simulink model "SF051A_SnsrOffsLrng"  (R2013b)
settings: Solver=FixedStepDiscrete  SolverMode=SingleTasking  StartTime=0.0  StopTime=1  FixedStep=0.002  RelTol=1e-3
undefined symbols (not defined in the file): ARCHGLBPRM_10MILLISEC_SEC_F32, ARCHGLBPRM_2MILLISEC_SEC_F32, ARCHGLBPRM_2PI_ULS_F32, ARCHGLBPRM_FLOATZEROTHD_ULS_F32, ARCHGLBPRM_PIOVER180_ULS_F32, CNV100MICROSECTOMILLISEC_MILLISECPERCNT_F32, CNV100MICROSECTOSEC_SECPERCNT_F32, COVRAMTRXNIT_ULS_F32, HWAUTHYTHD_ULS_F32, HWTQLRNGSTSLRND_CNT_U08, HWTQLRNGSTSNEGOFFS_CNT_U08, HWTQLRNGSTSNOTLRND_CNT_U08, HWTQLRNGSTSPOSOFFS_CNT_U08, HWTQLRNGSTSZEROOFFS_CNT_U08, HWTQLRNGTMRHILIM_SEC_F32, IDYMTRX_ULS_F32, IVS10MS_ULSPERSEC_F32, LRNGFILTICON_ULS_F32, NvmGetErrSts1, ONE_ULS_F32, SnsrOffsLrnd, SnsrOffsLrngFctEna, SnsrOffsLrngHwAgLrngDrvgDstThd, SnsrOffsLrngHwAgLrngEna, SnsrOffsLrngHwAgLrngHwVelThd, SnsrOffsLrngHwAgLrngSysTqThd, SnsrOffsLrngHwAgLrngSysTqThdMed, SnsrOffsLrngHwAgLrngSysTqThdTrustd, SnsrOffsLrngHwAgLrngSysTqThdWide, SnsrOffsLrngHwAgLrngTi, SnsrOffsLrngHwAgLrngVehSpdThd, SnsrOffsLrngHwAgLrngYawOffsDbnd, SnsrOffsLrngHwAgLrngYawRateThd, SnsrOffsLrngHwAgOffsLim, SnsrOffsLrngHwTqLrngEna, SnsrOffsLrngHwTqLrngEnaTiThd, SnsrOffsLrngHwTqLrngHwAgDbnd, SnsrOffsLrngHwTqLrngHwAgThd, SnsrOffsLrngHwTqLrngHwTqThd, SnsrOffsLrngHwTqLrngHwTqZeroOffsThd, SnsrOffsLrngHwTqLrngHwVelThd, SnsrOffsLrngHwTqLrngMeasTi, SnsrOffsLrngHwTqLrngMeasTiScar, SnsrOffsLrngHwTqLrngSampleImbThd1, SnsrOffsLrngHwTqLrngSampleImbThd2, SnsrOffsLrngHwTqLrngSampleThd1, SnsrOffsLrngHwTqLrngSampleThd2, SnsrOffsLrngHwTqLrngTiWghtCoeff, SnsrOffsLrngHwTqLrngVehSpdThd, SnsrOffsLrngHwTqOffsLim, SnsrOffsLrngSampleCntForHwTqLrngRst, SnsrOffsLrngTqInpDetnPwrEstimnThd, SnsrOffsLrngTqInpDetnSinGenrAmp, SnsrOffsLrngTqInpDetnSinGenrFrq, SnsrOffsLrngTqInpDetnStg1FilGain, SnsrOffsLrngTqInpDetnStg1WinSize, SnsrOffsLrngTqInpDetnStg2FilGainCen, SnsrOffsLrngTqInpDetnStg2FilGainDwn, SnsrOffsLrngTqInpDetnStg2FilGainUp, SnsrOffsLrngTqInpDetnStg2WinSize ... (+15)
libraries: Fil x34, FixdToFloat x17, FloatToFixd x16, NxtrLim x15, simulink x12, NxtrAbslt x12, NxtrNvM x8, NxtrMin x5, NxtrMath x3
(part 9 of 11)

== system SF051A_SnsrOffsLrng/SnsrOffsLrng/SnsrOffsLrngPer1/Learning/ForgettingFactor/ResetHwTqLrng/GetRefTmr100MicroSec32bit ==
  note: 1 count = 100 uSec
  note: seconds
  note: microseconds
  note: counts
  note: Wrap-to-zero
  note: GetRefTmr100MicroSec32bit
  note: Created Aug 18, 2015
      | Modified Oct 21, 2015
      | Modified Oct 30, 2015
      | Kevin Derry
  CopyRight2 : Subsystem  Description=|  mask(Copyright Information){none=on}
      | Copyright info block.                                               
      |                                                                     
      | Place copyright information at the top of every subsystem in design.
      mask prompts: none "No parameters"
      mask help: Place copyright information at the top of every subsystem in design.
      mask Display:
      | NxtrConf = 'Nexteer Confidential';
      | 
      | sys = bdroot; %handle for the current model ("system")
      | first = get_param(sys,'Created');
      | if(isempty(first))
      |     first = datestr(now,'yyyy');
      | else
      |     first = first(end-3:end);  %year is last four digits
      | end
      | 
      | last = get_param(sys,'LastModifiedDate');
      | if isempty(last)
      |     last = datestr(now,'yyyy');
      | else
      |     last = last(end-3:end);
      | end
      | 
      | if strcmp(first,last)
      |     fprintf('%s -- Copyright %s Nexteer',NxtrConf,first)
      | else
      |     fprintf('%s -- %s%s- %s Nexteer',NxtrConf,char(169),first,last)
      | end
  Count per uSec : Constant  Value=0.01
  Data Store Read1 : DataStoreRead  DataStoreName=SimnTi
  Data Type Conversion1 : DataTypeConversion  OutDataTypeStr=uint32
  Divide1 : Product  Inputs=**
  Divide2 : Product  Inputs=*/
  Max Counts : Constant  Value=2^32-1
  Product1 : Product
  Product2 : Product
  Rounding : Rounding
  Subtract1 : Sum  Inputs=+-
  uSec per Sec : Constant  Value=1000000
  RefTmr : Outport
  wires:
  Product2/1 -> Subtract1/2
  Subtract1/1 -> Data Type Conversion1/1
  Rounding/1 -> Product2/1
  Divide2/1 -> Rounding/1
  Max Counts/1 -> Divide2/2, Product2/2
  Divide1/1 -> Divide2/1, Subtract1/1
  Product1/1 -> Divide1/1
  Count per uSec/1 -> Divide1/2
  uSec per Sec/1 -> Product1/2
  Data Type Conversion1/1 -> RefTmr/1
  Data Store Read1/1 -> Product1/1

== system SF051A_SnsrOffsLrng/SnsrOffsLrng/SnsrOffsLrngPer1/Learning/ForgettingFactor/ResetHwTqLrng/Subsystem5 ==

== system SF051A_SnsrOffsLrng/SnsrOffsLrng/SnsrOffsLrngPer1/Learning/Recursive Least Square Regression/Calculate Covariance Matrix/Subsystem5 ==

== system SF051A_SnsrOffsLrng/SnsrOffsLrng/SnsrOffsLrngPer1/Learning/Recursive Least Square Regression/Calculate K Vector/Subsystem5 ==

== system SF051A_SnsrOffsLrng/SnsrOffsLrng/SnsrOffsLrngPer1/Learning/Recursive Least Square Regression/Update beta_k/Subsystem5 ==

== system SF051A_SnsrOffsLrng/SnsrOffsLrng/SnsrOffsLrngPer1/Learning/ValidityCheck/DecideOutputs/HwTrqNotLearnt ==
  Action Port : ActionPort  ActionType=else
  Constant1 : Constant  Value=false  OutDataTypeStr=boolean
      settings: AttributesFormatString=%<OutDataTypeStr>
  Constant3 : Constant  Value=HWTQLRNGSTSNOTLRND_CNT_U08  OutDataTypeStr=uint8
  Subsystem5 : Subsystem  Description=|  mask(Copyright Information){none=on}
      | Copyright info block.                                               
      |                                                                     
      | Place copyright information at the top of every subsystem in design.
      mask prompts: none "No parameters"
      mask help: Place copyright information at the top of every subsystem in design.
      mask Display:
      | NxtrConf = 'Nexteer Confidential';
      | 
      | sys = bdroot; %handle for the current model ("system")
      | first = get_param(sys,'Created');
      | first = first(end-3:end);  %year is last four digits
      | 
      | last = get_param(sys,'LastModifiedDate');
      | if isempty(last)
      |     last = datestr(now,'yyyy');
      | else
      |     last = last(end-3:end);
      | end
      | 
      | if strcmp(first,last)
      |     fprintf('%s -- Copyright %s Nexteer',NxtrConf,first)
      | else
      |     fprintf('%s -- %s%s- %s Nexteer',NxtrConf,char(169),first,last)
      | end
  LrngSts : Outport
  EstimnVld : Outport  Port=2
  wires:
  Constant3/1 -> LrngSts/1
  Constant1/1 -> EstimnVld/1

== system SF051A_SnsrOffsLrng/SnsrOffsLrng/SnsrOffsLrngPer1/Learning/ValidityCheck/DecideOutputs/HwTrqOffsetLearnt ==
  Action Port : ActionPort  ActionType=then
  Constant1 : Constant  Value=true  OutDataTypeStr=boolean
      settings: AttributesFormatString=%<OutDataTypeStr>
  Constant3 : Constant  Value=HWTQLRNGSTSLRND_CNT_U08  OutDataTypeStr=uint8
  Subsystem5 : Subsystem  Description=|  mask(Copyright Information){none=on}
      | Copyright info block.                                               
      |                                                                     
      | Place copyright information at the top of every subsystem in design.
      mask prompts: none "No parameters"
      mask help: Place copyright information at the top of every subsystem in design.
      mask Display:
      | NxtrConf = 'Nexteer Confidential';
      | 
      | sys = bdroot; %handle for the current model ("system")
      | first = get_param(sys,'Created');
      | first = first(end-3:end);  %year is last four digits
      | 
      | last = get_param(sys,'LastModifiedDate');
      | if isempty(last)
      |     last = datestr(now,'yyyy');
      | else
      |     last = last(end-3:end);
      | end
      | 
      | if strcmp(first,last)
      |     fprintf('%s -- Copyright %s Nexteer',NxtrConf,first)
      | else
      |     fprintf('%s -- %s%s- %s Nexteer',NxtrConf,char(169),first,last)
      | end
  LrngSts : Outport
  EstimnVld : Outport  Port=2
  wires:
  Constant1/1 -> EstimnVld/1
  Constant3/1 -> LrngSts/1

== system SF051A_SnsrOffsLrng/SnsrOffsLrng/SnsrOffsLrngPer1/Learning/ValidityCheck/DecideOutputs/Pos//Neg//Zero Offset Status Selector ==
  note: It selects the TOCStatus based on the value of the
      | estimated HwTrq Offset.
  note: TOCStatus
      | 0 = HwTrq NotLearned
      | 1 = Positive HwTrq Offset
      | 2 = Negative HwTrqOffset
      | 3 = Zero HwTrq Offset
      | 4 = HwTrq Offset Learned
  DriftEstimnOnCentr : Inport  RequirementInfo={'linktype_rmi_doors' '0000babd (/E-STEER Core/SubSystem Specifications/Application Functions/SF051A Sensor Offset Learning)' '#SF051A_186' 'true' 'REQ:SF051A_186' '' ; 'linktype_rmi_doors' '0000babd (/E-STEER Core/SubSystem Specifications/Application Functions/SF051A Sensor Offset Learning)' '#SF051A_195' 'true' 'REQ:SF051A_195' '' ; 'linktype_rmi_doors' '0000babd (/E-STEER Core/SubSystem Specifications/Application Functions/SF051A Sensor Offset Learning)' '#SF051A_194' 'true' 'REQ:SF051A_194' '' } %GIDa_29c46742_0190_4134_8ec7_44363e312a28
  Action Port : ActionPort  ActionType=elseif
  1_Positive HwTrq Offset : Subsystem  RequirementInfo={'linktype_rmi_doors' '0000babd (/E-STEER Core/SubSystem Specifications/Application Functions/SF051A Sensor Offset Learning)' '#SF051A_186' 'true' 'REQ:SF051A_186' '' } %GIDa_941a9e58_f1f3_40f2_8b3e_1b09aead3b41  TreatAsAtomicUnit=on
  2_Negative HwTrq Offset : Subsystem  RequirementInfo={'linktype_rmi_doors' '0000babd (/E-STEER Core/SubSystem Specifications/Application Functions/SF051A Sensor Offset Learning)' '#SF051A_195' 'true' 'REQ:SF051A_195' '' } %GIDa_c6d6cb28_240d_4435_ac45_3133f97fc59c  TreatAsAtomicUnit=on
  3_Zero HwTrq Offset : Subsystem  RequirementInfo={'linktype_rmi_doors' '0000babd (/E-STEER Core/SubSystem Specifications/Application Functions/SF051A Sensor Offset Learning)' '#SF051A_194' 'true' 'REQ:SF051A_194' '' } %GIDa_2db23fb9_9ed6_47ae_a299_df8f3702bd6f  TreatAsAtomicUnit=on
  Constant3 : Constant  Value=false  OutDataTypeStr=boolean
      settings: AttributesFormatString=%<OutDataTypeStr>
  Constant4 : Constant  RequirementInfo={'linktype_rmi_doors' '0000babd (/E-STEER Core/SubSystem Specifications/Application Functions/SF051A Sensor Offset Learning)' '#SF051A_186' 'true' 'REQ:SF051A_186' '' ; 'linktype_rmi_doors' '0000babd (/E-STEER Core/SubSystem Specifications/Application Functions/SF051A Sensor Offset Learning)' '#SF051A_195' 'true' 'REQ:SF051A_195' '' ; 'linktype_rmi_doors' '0000babd (/E-STEER Core/SubSystem Specifications/Application Functions/SF051A Sensor Offset Learning)' '#SF051A_194' 'true' 'REQ:SF051A_194' '' } %GIDa_0aa47765_2606_488c_aacb_fa125d44fe0b  Value=SnsrOffsLrngHwTqLrngHwTqZeroOffsThd
  If : If  RequirementInfo={'linktype_rmi_doors' '0000babd (/E-STEER Core/SubSystem Specifications/Application Functions/SF051A Sensor Offset Learning)' '#SF051A_186' 'true' 'REQ:SF051A_186' '' ; 'linktype_rmi_doors' '0000babd (/E-STEER Core/SubSystem Specifications/Application Functions/SF051A Sensor Offset Learning)' '#SF051A_195' 'true' 'REQ:SF051A_195' '' ; 'linktype_rmi_doors' '0000babd (/E-STEER Core/SubSystem Specifications/Application Functions/SF051A Sensor Offset Learning)' '#SF051A_194' 'true' 'REQ:SF051A_194' '' } %GIDa_36d740f7_db76_41fe_83e8_1901bd872b17  NumInputs=2  IfExpression=u1  ElseIfExpressions=u2
  Merge : Merge  Inputs=3
  Relational Operator : RelationalOperator  RequirementInfo={'linktype_rmi_doors' '0000babd (/E-STEER Core/SubSystem Specifications/Application Functions/SF051A Sensor Offset Learning)' '#SF051A_186' 'true' 'REQ:SF051A_186' '' ; 'linktype_rmi_doors' '0000babd (/E-STEER Core/SubSystem Specifications/Application Functions/SF051A Sensor Offset Learning)' '#SF051A_195' 'true' 'REQ:SF051A_195' '' ; 'linktype_rmi_doors' '0000babd (/E-STEER Core/SubSystem Specifications/Application Functions/SF051A Sensor Offset Learning)' '#SF051A_194' 'true' 'REQ:SF051A_194' '' } %GIDa_6b1f25fd_0620_4f2d_83a5_fa63c4ad4805  Operator=>  OutDataTypeStr=boolean
  Relational Operator1 : RelationalOperator  RequirementInfo={'linktype_rmi_doors' '0000babd (/E-STEER Core/SubSystem Specifications/Application Functions/SF051A Sensor Offset Learning)' '#SF051A_186' 'true' 'REQ:SF051A_186' '' ; 'linktype_rmi_doors' '0000babd (/E-STEER Core/SubSystem Specifications/Application Functions/SF051A Sensor Offset Learning)' '#SF051A_195' 'true' 'REQ:SF051A_195' '' ; 'linktype_rmi_doors' '0000babd (/E-STEER Core/SubSystem Specifications/Application Functions/SF051A Sensor Offset Learning)' '#SF051A_194' 'true' 'REQ:SF051A_194' '' } %GIDa_895639c2_4ad1_4cae_b7c9_5da33bf76dd8  Operator=<  OutDataTypeStr=boolean
  Subsystem5 : Subsystem  Description=|  mask(Copyright Information){none=on}
      | Copyright info block.                                               
      |                                                                     
      | Place copyright information at the top of every subsystem in design.
      mask prompts: none "No parameters"
      mask help: Place copyright information at the top of every subsystem in design.
      mask Display:
      | NxtrConf = 'Nexteer Confidential';
      | 
      | sys = bdroot; %handle for the current model ("system")
      | first = get_param(sys,'Created');
      | first = first(end-3:end);  %year is last four digits
      | 
      | last = get_param(sys,'LastModifiedDate');
      | if isempty(last)
      |     last = datestr(now,'yyyy');
      | else
      |     last = last(end-3:end);
      | end
      | 
      | if strcmp(first,last)
      |     fprintf('%s -- Copyright %s Nexteer',NxtrConf,first)
      | else
      |     fprintf('%s -- %s%s- %s Nexteer',NxtrConf,char(169),first,last)
      | end
  Unary Minus : UnaryMinus  RequirementInfo={'linktype_rmi_doors' '0000babd (/E-STEER Core/SubSystem Specifications/Application Functions/SF051A Sensor Offset Learning)' '#SF051A_186' 'true' 'REQ:SF051A_186' '' ; 'linktype_rmi_doors' '0000babd (/E-STEER Core/SubSystem Specifications/Application Functions/SF051A Sensor Offset Learning)' '#SF051A_195' 'true' 'REQ:SF051A_195' '' ; 'linktype_rmi_doors' '0000babd (/E-STEER Core/SubSystem Specifications/Application Functions/SF051A Sensor Offset Learning)' '#SF051A_194' 'true' 'REQ:SF051A_194' '' } %GIDa_b390a6a0_37ce_48b2_968e_7797d0461aea
  LrngSts : Outport
  EstimnVld : Outport  Port=2
  wires:
  1_Positive HwTrq Offset/1(TOCStatus) -> Merge/1
  If/2 -> 2_Negative HwTrq Offset/Action
  If/3 -> 3_Zero HwTrq Offset/Action
  2_Negative HwTrq Offset/1(TOCStatus) -> Merge/2
  3_Zero HwTrq Offset/1(TOCStatus) -> Merge/3
  If/1 -> 1_Positive HwTrq Offset/Action
  Constant3/1 -> EstimnVld/1
  Constant4/1 -> Relational Operator/2, Unary Minus/1
  Merge/1 -> LrngSts/1
  Unary Minus/1 -> Relational Operator1/2
  [DriftEstimnOnCentr] -> Relational Operator1/1
  DriftEstimnOnCentr/1 -> Relational Operator/1, [DriftEstimnOnCentr]
  Relational Operator1/1 -> If/2
  Relational Operator/1 -> If/1

== system SF051A_SnsrOffsLrng/SnsrOffsLrng/SnsrOffsLrngPer1/Learning/ValidityCheck/DecideOutputs/Subsystem5 ==

== system SF051A_SnsrOffsLrng/SnsrOffsLrng/SnsrOffsLrngPer1/Learning/ValidityCheck/HwTrqNotLearnt/Subsystem5 ==

== system SF051A_SnsrOffsLrng/SnsrOffsLrng/SnsrOffsLrngPer1/Measurements_Grabber/GetTiSpan100MicroSec32bit/No wrapping/CopyRight2 ==

== system SF051A_SnsrOffsLrng/SnsrOffsLrng/SnsrOffsLrngPer1/Measurements_Grabber/GetTiSpan100MicroSec32bit/Wrapping/CopyRight2 ==

== system SF051A_SnsrOffsLrng/SnsrOffsLrng/SnsrOffsLrngPer1/Measurements_Grabber/True_UpdateNVMRam/GetRefTmr100MicroSec32bit/CopyRight2 ==

== system SF051A_SnsrOffsLrng/SnsrOffsLrng/SnsrOffsLrngPer2/Enable_Function/POC/Do nothing/Subsystem5 ==

== system SF051A_SnsrOffsLrng/SnsrOffsLrng/SnsrOffsLrngPer2/Enable_Function/POC/Do nothing1/Subsystem5 ==

== system SF051A_SnsrOffsLrng/SnsrOffsLrng/SnsrOffsLrngPer2/Enable_Function/POC/Learn/BiasEstimation_ValidityCheck ==
  note: This "if" was reordered to avoid coverage issues. No functional impact.
  HwTqLrngSts : Inport
  ElpsdTi : Inport  Port=2
  HwPosBiasEstRaw : Inport  Port=3
  SysTqAvrg : Inport  Port=4
  Do nothing : Subsystem  TreatAsAtomicUnit=on
  HwTqAvrg_Check : Subsystem  RequirementInfo={'linktype_rmi_doors' '0000babd (/E-STEER Core/SubSystem Specifications/Application Functions/SF051A Sensor Offset Learning)' '#SF051A_115' 'true' 'REQ:SF051A_115' '' } %GIDa_ee7508ac_a4c4_4f2e_8fb0_f0302cd0680f
  If1 : If  IfExpression=u1
  Keep OR Reset : Subsystem
  Subsystem5 : Subsystem  Description=|  mask(Copyright Information){none=on}
      | Copyright info block.                                               
      |                                                                     
      | Place copyright information at the top of every subsystem in design.
      mask prompts: none "No parameters"
      mask help: Place copyright information at the top of every subsystem in design.
      mask Display:
      | NxtrConf = 'Nexteer Confidential';
      | 
      | sys = bdroot; %handle for the current model ("system")
      | first = get_param(sys,'Created');
      | first = first(end-3:end);  %year is last four digits
      | 
      | last = get_param(sys,'LastModifiedDate');
      | if isempty(last)
      |     last = datestr(now,'yyyy');
      | else
      |     last = last(end-3:end);
      | end
      | 
      | if strcmp(first,last)
      |     fprintf('%s -- Copyright %s Nexteer',NxtrConf,first)
      | else
      |     fprintf('%s -- %s%s- %s Nexteer',NxtrConf,char(169),first,last)
      | end
  Time_Check : Subsystem
  wires:
  SysTqAvrg/1 -> HwTqAvrg_Check/1(SysTqAvrg)
  ElpsdTi/1 -> Time_Check/1(ElpsdTi)
  Time_Check/1(TiVldFlg) -> If1/1
  HwTqLrngSts/1 -> HwTqAvrg_Check/2(HwTqLrngSts)
  If1/2 -> Do nothing/Action
  HwPosBiasEstRaw/1 -> Keep OR Reset/1(HwPosBiasEstRaw)
  HwTqAvrg_Check/1(TqVldFlg) -> Keep OR Reset/2(TqVldFlg)
  If1/1 -> Keep OR Reset/Action

== system SF051A_SnsrOffsLrng/SnsrOffsLrng/SnsrOffsLrngPer2/Enable_Function/POC/Learn/LPFs ==
  note: Apply slow filters to Driver + Assist Torque. After tunable period of time, this will be used to decide whether the road was flat and wind was calm (or at least averaged themselves out over the time period).
  note: Same fc for both paths
  note: Two LPF in series to achieve a less noisy estimation
  HwAgFild : Inport
  SysTqFild : Inport  Port=2
  Add1 : Sum  RequirementInfo={'linktype_rmi_doors' '0000babd (/E-STEER Core/SubSystem Specifications/Application Functions/SF051A Sensor Offset Learning)' '#SF051A_118' 'true' 'REQ:SF051A_118' '' } %GIDa_a9eb681f_cac0_43af_beb2_f1f51fe05355
  FilLpUpdOutp : Fil/FilLpUpdOutp  RequirementInfo={'linktype_rmi_doors' '0000babd (/E-STEER Core/SubSystem Specifications/Application Functions/SF051A Sensor Offset Learning)' '#SF051A_120' 'true' 'REQ:SF051A_120' '' } %GIDa_e30aba0f_56bd_4fdb_8776_c681c8d8de47  StVar=HwAgLrngFil1
      settings: AttributesFormatString=StVar: %<StVar>
  FilLpUpdOutp1 : Fil/FilLpUpdOutp  RequirementInfo={'linktype_rmi_doors' '0000babd (/E-STEER Core/SubSystem Specifications/Application Functions/SF051A Sensor Offset Learning)' '#SF051A_120' 'true' 'REQ:SF051A_120' '' } %GIDa_e1bf3bcc_7598_44e1_9e26_8397d90c3eeb  StVar=HwAgLrngFil2
      settings: AttributesFormatString=StVar: %<StVar>
  FilLpUpdOutp2 : Fil/FilLpUpdOutp  RequirementInfo={'linktype_rmi_doors' '0000babd (/E-STEER Core/SubSystem Specifications/Application Functions/SF051A Sensor Offset Learning)' '#SF051A_116' 'true' 'REQ:SF051A_116' '' } %GIDa_0425a662_6a46_4ec4_80ca_4f7f05c68403  StVar=HwAgLrngSysTqFil1
      settings: AttributesFormatString=StVar: %<StVar>
  FilLpUpdOutp3 : Fil/FilLpUpdOutp  RequirementInfo={'linktype_rmi_doors' '0000babd (/E-STEER Core/SubSystem Specifications/Application Functions/SF051A Sensor Offset Learning)' '#SF051A_116' 'true' 'REQ:SF051A_116' '' } %GIDa_d241de31_ede3_4c71_a352_ed2f5f77ad04  StVar=HwAgLrngSysTqFil2
      settings: AttributesFormatString=StVar: %<StVar>
  FloatToFixd_s16_f1 : FloatToFixd/FloatToFixd_s16_f32  Param1=5
  FloatToFixd_s16_f32 : FloatToFixd/FloatToFixd_s16_f32  Param1=4
  NvmRam : DataStoreWrite  RequirementInfo={'linktype_rmi_doors' '0000babd (/E-STEER Core/SubSystem Specifications/Application Functions/SF051A Sensor Offset Learning)' '#SF051A_119' 'true' 'REQ:SF051A_119' '' } %GIDa_7d3fe29f_62c5_41ed_8a64_f23320f0f4e5  DataStoreName=SnsrOffsLrnd  DataStoreElements=SnsrOffsLrnd.HwAgLrngHwAgFilSt#SnsrOffsLrnd.HwAgLrngSysTqFilSt
  Read NVMRam : DataStoreRead  RequirementInfo={'linktype_rmi_doors' '0000babd (/E-STEER Core/SubSystem Specifications/Application Functions/SF051A Sensor Offset Learning)' '#SF051A_118' 'true' 'REQ:SF051A_118' '' } %GIDa_3e1188c8_61c6_4a14_9b93_b71b1baf8e86  DataStoreName=SnsrOffsLrnd  DataStoreElements=SnsrOffsLrnd.HwAgLrndTi
  Subsystem5 : Subsystem  Description=|  mask(Copyright Information){none=on}
      | Copyright info block.                                               
      |                                                                     
      | Place copyright information at the top of every subsystem in design.
      mask prompts: none "No parameters"
      mask help: Place copyright information at the top of every subsystem in design.
      mask Display:
      | NxtrConf = 'Nexteer Confidential';
      | 
      | sys = bdroot; %handle for the current model ("system")
      | first = get_param(sys,'Created');
      | first = first(end-3:end);  %year is last four digits
      | 
      | last = get_param(sys,'LastModifiedDate');
      | if isempty(last)
      |     last = datestr(now,'yyyy');
      | else
      |     last = last(end-3:end);
      | end
      | 
      | if strcmp(first,last)
      |     fprintf('%s -- Copyright %s Nexteer',NxtrConf,first)
      | else
      |     fprintf('%s -- %s%s- %s Nexteer',NxtrConf,char(169),first,last)
      | end
  Ts : Constant  RequirementInfo={'linktype_rmi_doors' '0000babd (/E-STEER Core/SubSystem Specifications/Application Functions/SF051A Sensor Offset Learning)' '#SF051A_118' 'true' 'REQ:SF051A_118' '' } %GIDa_d54cb801_cb5c_4254_a813_9ff94058f6aa  Value=ARCHGLBPRM_10MILLISEC_SEC_F32
  ElpsdTi : Outport  OutDataTypeStr=single
  HwPosBiasEstRaw : Outport  Port=2
  SysTqAvrg : Outport  RequirementInfo={'linktype_rmi_doors' '0000babd (/E-STEER Core/SubSystem Specifications/Application Functions/SF051A Sensor Offset Learning)' '#SF051A_116' 'true' 'REQ:SF051A_116' '' } %GIDa_b3eceb47_afae_4bf7_8f18_e381e2b43915  Port=3
  wires:
  HwAgFild/1 -> FilLpUpdOutp/1
  FilLpUpdOutp1/1 -> FloatToFixd_s16_f32/1, HwPosBiasEstRaw/1
  SysTqFild/1 -> FilLpUpdOutp2/1
  FilLpUpdOutp3/1 -> FloatToFixd_s16_f1/1, SysTqAvrg/1
  Read NVMRam/1 -> Add1/1
  Ts/1 -> Add1/2
  Add1/1 -> ElpsdTi/1  "ElpsdTi"
  FloatToFixd_s16_f32/1 -> NvmRam/1
  FloatToFixd_s16_f1/1 -> NvmRam/2
  FilLpUpdOutp/1 -> FilLpUpdOutp1/1
  FilLpUpdOutp2/1 -> FilLpUpdOutp3/1

== system SF051A_SnsrOffsLrng/SnsrOffsLrng/SnsrOffsLrngPer2/Enable_Function/POC/Learn/Subsystem5 ==

== system SF051A_SnsrOffsLrng/SnsrOffsLrng/SnsrOffsLrngPer2/Enable_Function/POC/Learning Conditions/DrivingStraight ==
  note: Calculate distance travelled. Learning conditions must be true for a minimum driving distance before learning begins.
  VehSpd : Inport  OutDataTypeStr=single
  Action Port : ActionPort  ActionType=then
  Constant : Constant  Value=ARCHGLBPRM_10MILLISEC_SEC_F32
  Constant1 : Constant  Value=SPDCNVN_MTRPERSECPERKPH_F32
  Data Store Read : DataStoreRead  DataStoreName=HwAgLrngDrvgDstPrev
  LimStat_f32 : NxtrLim/LimStat_f32  LoLim=ZERO_ULS_F32  HiLim=SnsrOffsLrngHwAgLrngDrvgDstThd
      settings: AttributesFormatString=|
      | Low Limit: %<LoLim>
      | High Limit:%<HiLim>
  Product : Product  Inputs=3  OutDataTypeStr=single  RndMeth=Zero
  Subsystem5 : Subsystem  Description=|  mask(Copyright Information){none=on}
      | Copyright info block.                                               
      |                                                                     
      | Place copyright information at the top of every subsystem in design.
      mask prompts: none "No parameters"
      mask help: Place copyright information at the top of every subsystem in design.
      mask Display:
      | NxtrConf = 'Nexteer Confidential';
      | 
      | sys = bdroot; %handle for the current model ("system")
      | first = get_param(sys,'Created');
      | first = first(end-3:end);  %year is last four digits
      | 
      | last = get_param(sys,'LastModifiedDate');
      | if isempty(last)
      |     last = datestr(now,'yyyy');
      | else
      |     last = last(end-3:end);
      | end
      | 
      | if strcmp(first,last)
      |     fprintf('%s -- Copyright %s Nexteer',NxtrConf,first)
      | else
      |     fprintf('%s -- %s%s- %s Nexteer',NxtrConf,char(169),first,last)
      | end
  Sum : Sum
  HwAgLrngDrvgDst : Outport
  wires:
  Product/1 -> Sum/1
  Constant/1 -> Product/3
  VehSpd/1 -> Product/1
  Sum/1 -> LimStat_f32/1
  Constant1/1 -> Product/2
  Data Store Read/1 -> Sum/2
  LimStat_f32/1 -> HwAgLrngDrvgDst/1

== system SF051A_SnsrOffsLrng/SnsrOffsLrng/SnsrOffsLrngPer2/Enable_Function/POC/Learning Conditions/NotDrivingStraight ==
  Action Port : ActionPort  ActionType=else
  DistanceTravelled : Constant  Value=ZERO_ULS_F32  OutDataTypeStr=single
      settings: AttributesFormatString=%<OutDataTypeStr>
  Subsystem5 : Subsystem  Description=|  mask(Copyright Information){none=on}
      | Copyright info block.                                               
      |                                                                     
      | Place copyright information at the top of every subsystem in design.
      mask prompts: none "No parameters"
      mask help: Place copyright information at the top of every subsystem in design.
      mask Display:
      | NxtrConf = 'Nexteer Confidential';
      | 
      | sys = bdroot; %handle for the current model ("system")
      | first = get_param(sys,'Created');
      | first = first(end-3:end);  %year is last four digits
      | 
      | last = get_param(sys,'LastModifiedDate');
      | if isempty(last)
      |     last = datestr(now,'yyyy');
      | else
      |     last = last(end-3:end);
      | end
      | 
      | if strcmp(first,last)
      |     fprintf('%s -- Copyright %s Nexteer',NxtrConf,first)
      | else
      |     fprintf('%s -- %s%s- %s Nexteer',NxtrConf,char(169),first,last)
      | end
  HwAgLrngDrvgDstPrev : Outport
  wires:
  DistanceTravelled/1 -> HwAgLrngDrvgDstPrev/1

== system SF051A_SnsrOffsLrng/SnsrOffsLrng/SnsrOffsLrngPer2/Enable_Function/POC/Learning Conditions/Subsystem5 ==

== system SF051A_SnsrOffsLrng/SnsrOffsLrng/SnsrOffsLrngPer2/Enable_Function/POC/Reset_HwAg_Learning/Subsystem5 ==

== system SF051A_SnsrOffsLrng/SnsrOffsLrng/SnsrOffsLrngPer2/Enable_Function/SOaC_HierarchyManager/POCEnabler/Subsystem5 ==

== system SF051A_SnsrOffsLrng/SnsrOffsLrng/SnsrOffsLrngPer2/Enable_Function/SOaC_HierarchyManager/POCResetLogic/Subsystem5 ==

== system SF051A_SnsrOffsLrng/SnsrOffsLrng/SnsrOffsLrngPer2/Enable_Function/SOaC_HierarchyManager/YOCEnabler/Subsystem5 ==

== system SF051A_SnsrOffsLrng/SnsrOffsLrng/SnsrOffsLrngPer2/Enable_Function/YOC/Do nothing/Subsystem5 ==

== system SF051A_SnsrOffsLrng/SnsrOffsLrng/SnsrOffsLrngPer2/Enable_Function/YOC/Learn/Do nothing ==
  Action Port : ActionPort  ActionType=else
  Subsystem5 : Subsystem  Description=|  mask(Copyright Information){none=on}
      | Copyright info block.                                               
      |                                                                     
      | Place copyright information at the top of every subsystem in design.
      mask prompts: none "No parameters"
      mask help: Place copyright information at the top of every subsystem in design.
      mask Display:
      | NxtrConf = 'Nexteer Confidential';
      | 
      | sys = bdroot; %handle for the current model ("system")
      | first = get_param(sys,'Created');
      | first = first(end-3:end);  %year is last four digits
      | 
      | last = get_param(sys,'LastModifiedDate');
      | if isempty(last)
      |     last = datestr(now,'yyyy');
      | else
      |     last = last(end-3:end);
      | end
      | 
      | if strcmp(first,last)
      |     fprintf('%s -- Copyright %s Nexteer',NxtrConf,first)
      | else
      |     fprintf('%s -- %s%s- %s Nexteer',NxtrConf,char(169),first,last)
      | end

== system SF051A_SnsrOffsLrng/SnsrOffsLrng/SnsrOffsLrngPer2/Enable_Function/YOC/Learn/Filter For Learning ==
  note: Two LPF in series to achieve a less noisy estimation
  YawRate : Inport
  Display : DataStoreWrite  DataStoreName=dSnsrOffsLrngYawLrngBiasEstimnRaw
  FilLpUpdOutp : Fil/FilLpUpdOutp  RequirementInfo={'linktype_rmi_doors' '0000babd (/E-STEER Core/SubSystem Specifications/Application Functions/SF051A Sensor Offset Learning)' '#SF051A_91' 'true' 'REQ:SF051A_91' '' } %GIDa_e675741c_4393_4ae0_8c11_3d9c4cd73306  StVar=YawLrngFil1
      settings: AttributesFormatString=StVar: %<StVar>
  FilLpUpdOutp1 : Fil/FilLpUpdOutp  RequirementInfo={'linktype_rmi_doors' '0000babd (/E-STEER Core/SubSystem Specifications/Application Functions/SF051A Sensor Offset Learning)' '#SF051A_91' 'true' 'REQ:SF051A_91' '' } %GIDa_c1158e21_cba4_48b8_986e_44a0cef26229  StVar=YawLrngFil2
      settings: AttributesFormatString=StVar: %<StVar>
  Subsystem5 : Subsystem  Description=|  mask(Copyright Information){none=on}
      | Copyright info block.                                               
      |                                                                     
      | Place copyright information at the top of every subsystem in design.
      mask prompts: none "No parameters"
      mask help: Place copyright information at the top of every subsystem in design.
      mask Display:
      | NxtrConf = 'Nexteer Confidential';
      | 
      | sys = bdroot; %handle for the current model ("system")
      | first = get_param(sys,'Created');
      | first = first(end-3:end);  %year is last four digits
      | 
      | last = get_param(sys,'LastModifiedDate');
      | if isempty(last)
      |     last = datestr(now,'yyyy');
      | else
      |     last = last(end-3:end);
      | end
      | 
      | if strcmp(first,last)
      |     fprintf('%s -- Copyright %s Nexteer',NxtrConf,first)
      | else
      |     fprintf('%s -- %s%s- %s Nexteer',NxtrConf,char(169),first,last)
      | end
  LrndBias : Outport
  wires:
  YawRate/1 -> FilLpUpdOutp/1
  FilLpUpdOutp1/1 -> Display/1, LrndBias/1
  FilLpUpdOutp/1 -> FilLpUpdOutp1/1

== system SF051A_SnsrOffsLrng/SnsrOffsLrng/SnsrOffsLrngPer2/Enable_Function/YOC/Learn/Subsystem5 ==

== system SF051A_SnsrOffsLrng/SnsrOffsLrng/SnsrOffsLrngPer2/Enable_Function/YOC/Learn/Update NVM RAM ==
  LrndBias : Inport
  Action Port : ActionPort  ActionType=then
  Constant1 : Constant  RequirementInfo={'linktype_rmi_doors' '0000babd (/E-STEER Core/SubSystem Specifications/Application Functions/SF051A Sensor Offset Learning)' '#SF051A_106' 'true' 'REQ:SF051A_106' '' } %GIDa_37485109_fb46_48dc_909d_b521f071c2b9  Value=SnsrOffsLrngYawRateOffsLim  OutDataTypeStr=single
  Constant3 : Constant  Value=ZERO_ULS_F32  OutDataTypeStr=single
      settings: AttributesFormatString=%<OutDataTypeStr>
  Constant4 : Constant  RequirementInfo={'linktype_rmi_doors' '0000babd (/E-STEER Core/SubSystem Specifications/Application Functions/SF051A Sensor Offset Learning)' '#SF051A_105' 'true' 'REQ:SF051A_105' '' ; 'linktype_rmi_doors' '0000babd (/E-STEER Core/SubSystem Specifications/Application Functions/SF051A Sensor Offset Learning)' '#SF051A_104' 'true' 'REQ:SF051A_104' '' } %GIDa_df24ee46_4669_4b46_bb68_420380373386  Value=true  OutDataTypeStr=boolean
      settings: AttributesFormatString=%<OutDataTypeStr>
  FloatToFixd_s16_f32 : FloatToFixd/FloatToFixd_s16_f32  Param1=9
  LimDyn_f32 : NxtrLim/LimDyn_f32  RequirementInfo={'linktype_rmi_doors' '0000babd (/E-STEER Core/SubSystem Specifications/Application Functions/SF051A Sensor Offset Learning)' '#SF051A_106' 'true' 'REQ:SF051A_106' '' } %GIDa_6d1d6713_3cf4_46d4_89d3_eaae33798d40
  Subsystem5 : Subsystem  Description=|  mask(Copyright Information){none=on}
      | Copyright info block.                                               
      |                                                                     
      | Place copyright information at the top of every subsystem in design.
      mask prompts: none "No parameters"
      mask help: Place copyright information at the top of every subsystem in design.
      mask Display:
      | NxtrConf = 'Nexteer Confidential';
      | 
      | sys = bdroot; %handle for the current model ("system")
      | first = get_param(sys,'Created');
      | first = first(end-3:end);  %year is last four digits
      | 
      | last = get_param(sys,'LastModifiedDate');
      | if isempty(last)
      |     last = datestr(now,'yyyy');
      | else
      |     last = last(end-3:end);
      | end
      | 
      | if strcmp(first,last)
      |     fprintf('%s -- Copyright %s Nexteer',NxtrConf,first)
      | else
      |     fprintf('%s -- %s%s- %s Nexteer',NxtrConf,char(169),first,last)
      | end
  Unary Minus : UnaryMinus  RequirementInfo={'linktype_rmi_doors' '0000babd (/E-STEER Core/SubSystem Specifications/Application Functions/SF051A Sensor Offset Learning)' '#SF051A_106' 'true' 'REQ:SF051A_106' '' } %GIDa_a9a854f0_810d_4d5e_9ca1_adb6c6a73d36
  Update NVM RAM1 : DataStoreWrite  RequirementInfo={'linktype_rmi_doors' '0000babd (/E-STEER Core/SubSystem Specifications/Application Functions/SF051A Sensor Offset Learning)' '#SF051A_91' 'true' 'REQ:SF051A_91' '' ; 'linktype_rmi_doors' '0000babd (/E-STEER Core/SubSystem Specifications/Application Functions/SF051A Sensor Offset Learning)' '#SF051A_240' 'true' 'REQ:SF051A_240' '' } %GIDa_01821431_abd4_4c49_acc0_aea480f79169  DataStoreName=SnsrOffsLrnd  DataStoreElements=SnsrOffsLrnd.YawRateOffs#SnsrOffsLrnd.YawRateOffsVld#SnsrOffsLrnd.YawRateElpdTi
  wires:
  LrndBias/1 -> LimDyn_f32/1
  Constant1/1 -> LimDyn_f32/3, Unary Minus/1
  Unary Minus/1 -> LimDyn_f32/2
  LimDyn_f32/1 -> FloatToFixd_s16_f32/1
  Constant3/1 -> Update NVM RAM1/3
  Constant4/1 -> Update NVM RAM1/2
  FloatToFixd_s16_f32/1 -> Update NVM RAM1/1

== system SF051A_SnsrOffsLrng/SnsrOffsLrng/SnsrOffsLrngPer2/Enable_Function/YOC/Learning Conditions/Subsystem5 ==

== system SF051A_SnsrOffsLrng/SnsrOffsLrng/SnsrOffsLrngPer1/EnableLearning/EnablingConditions/CheckLastMeasHwPos/FalseOut_KeepRef/Subsystem5 ==

== system SF051A_SnsrOffsLrng/SnsrOffsLrng/SnsrOffsLrngPer1/EnableLearning/EnablingConditions/CheckLastMeasHwPos/TrueOut_ResetRef/Subsystem5 ==

== system SF051A_SnsrOffsLrng/SnsrOffsLrng/SnsrOffsLrngPer1/EnableLearning/Eval_Time/GetTiSpan100MicroSec32bit/No wrapping/CopyRight2 ==

== system SF051A_SnsrOffsLrng/SnsrOffsLrng/SnsrOffsLrngPer1/EnableLearning/Eval_Time/GetTiSpan100MicroSec32bit/Wrapping/CopyRight2 ==

== system SF051A_SnsrOffsLrng/SnsrOffsLrng/SnsrOffsLrngPer1/EnableLearning/Perform_TqInpDetn/Enable_PreProcessing/False_Hold/Subsystem5 ==

== system SF051A_SnsrOffsLrng/SnsrOffsLrng/SnsrOffsLrngPer1/EnableLearning/Perform_TqInpDetn/Enable_PreProcessing/If Action Subsystem/Subsystem5 ==

== system SF051A_SnsrOffsLrng/SnsrOffsLrng/SnsrOffsLrngPer1/EnableLearning/Perform_TqInpDetn/Enable_PreProcessing/If Action Subsystem/True_False ==
  Action Port : ActionPort  ActionType=else
  Constant : Constant  Value=true  OutDataTypeStr=boolean
      settings: AttributesFormatString=%<OutDataTypeStr>
  Constant1 : Constant  Value=false  OutDataTypeStr=boolean
      settings: AttributesFormatString=%<OutDataTypeStr>
  Subsystem5 : Subsystem  Description=|  mask(Copyright Information){none=on}
      | Copyright info block.                                               
      |                                                                     
      | Place copyright information at the top of every subsystem in design.
      mask prompts: none "No parameters"
      mask help: Place copyright information at the top of every subsystem in design.
      mask Display:
      | NxtrConf = 'Nexteer Confidential';
      | 
      | sys = bdroot; %handle for the current model ("system")
      | first = get_param(sys,'Created');
      | first = first(end-3:end);  %year is last four digits
      | 
      | last = get_param(sys,'LastModifiedDate');
      | if isempty(last)
      |     last = datestr(now,'yyyy');
      | else
      |     last = last(end-3:end);
      | end
      | 
      | if strcmp(first,last)
      |     fprintf('%s -- Copyright %s Nexteer',NxtrConf,first)
      | else
      |     fprintf('%s -- %s%s- %s Nexteer',NxtrConf,char(169),first,last)
      | end
  Vld : Outport
  Prsnt : Outport  Port=2
  wires:
  Constant/1 -> Vld/1
  Constant1/1 -> Prsnt/1

== system SF051A_SnsrOffsLrng/SnsrOffsLrng/SnsrOffsLrngPer1/EnableLearning/Perform_TqInpDetn/Enable_PreProcessing/If Action Subsystem/True_True ==
  Action Port : ActionPort  ActionType=then
  Constant : Constant  Value=true  OutDataTypeStr=boolean
      settings: AttributesFormatString=%<OutDataTypeStr>
  Constant1 : Constant  Value=true  OutDataTypeStr=boolean
      settings: AttributesFormatString=%<OutDataTypeStr>
  Subsystem5 : Subsystem  Description=|  mask(Copyright Information){none=on}
      | Copyright info block.                                               
      |                                                                     
      | Place copyright information at the top of every subsystem in design.
      mask prompts: none "No parameters"
      mask help: Place copyright information at the top of every subsystem in design.
      mask Display:
      | NxtrConf = 'Nexteer Confidential';
      | 
      | sys = bdroot; %handle for the current model ("system")
      | first = get_param(sys,'Created');
      | first = first(end-3:end);  %year is last four digits
      | 
      | last = get_param(sys,'LastModifiedDate');
      | if isempty(last)
      |     last = datestr(now,'yyyy');
      | else
      |     last = last(end-3:end);
      | end
      | 
      | if strcmp(first,last)
      |     fprintf('%s -- Copyright %s Nexteer',NxtrConf,first)
      | else
      |     fprintf('%s -- %s%s- %s Nexteer',NxtrConf,char(169),first,last)
      | end
  Vld : Outport
  Prsnt : Outport  Port=2
  wires:
  Constant/1 -> Vld/1
  Constant1/1 -> Prsnt/1

== system SF051A_SnsrOffsLrng/SnsrOffsLrng/SnsrOffsLrngPer1/EnableLearning/Perform_TqInpDetn/Enable_PreProcessing/Preprocessing/Do nothing ==
  Action Port : ActionPort  ActionType=else
  Subsystem5 : Subsystem  Description=|  mask(Copyright Information){none=on}
      | Copyright info block.                                               
      |                                                                     
      | Place copyright information at the top of every subsystem in design.
      mask prompts: none "No parameters"
      mask help: Place copyright information at the top of every subsystem in design.
      mask Display:
      | NxtrConf = 'Nexteer Confidential';
      | 
      | sys = bdroot; %handle for the current model ("system")
      | first = get_param(sys,'Created');
      | first = first(end-3:end);  %year is last four digits
      | 
      | last = get_param(sys,'LastModifiedDate');
      | if isempty(last)
      |     last = datestr(now,'yyyy');
      | else
      |     last = last(end-3:end);
      | end
      | 
      | if strcmp(first,last)
      |     fprintf('%s -- Copyright %s Nexteer',NxtrConf,first)
      | else
      |     fprintf('%s -- %s%s- %s Nexteer',NxtrConf,char(169),first,last)
      | end

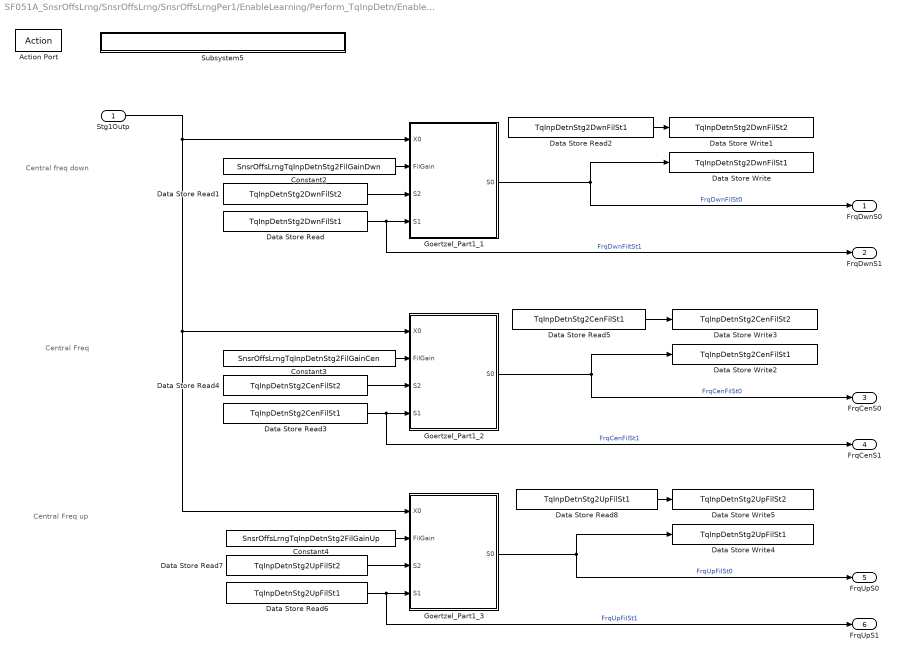
== system SF051A_SnsrOffsLrng/SnsrOffsLrng/SnsrOffsLrngPer1/EnableLearning/Perform_TqInpDetn/Enable_PreProcessing/Preprocessing/General_Goertzel ==
  note: Central Freq
  note: Central freq down
  note: Central Freq up
  Stg1Outp : Inport  OutDataTypeStr=single
  Action Port : ActionPort  ActionType=then
  Constant2 : Constant  Value=SnsrOffsLrngTqInpDetnStg2FilGainDwn
  Constant3 : Constant  Value=SnsrOffsLrngTqInpDetnStg2FilGainCen
  Constant4 : Constant  Value=SnsrOffsLrngTqInpDetnStg2FilGainUp
  Data Store Read : DataStoreRead  Priority=1  DataStoreName=TqInpDetnStg2DwnFilSt1
      settings: AttributesFormatString=priority: %<Priority>
  Data Store Read1 : DataStoreRead  Priority=1  DataStoreName=TqInpDetnStg2DwnFilSt2
  Data Store Read2 : DataStoreRead  Priority=2  DataStoreName=TqInpDetnStg2DwnFilSt1
      settings: AttributesFormatString=priority: %<Priority>
  Data Store Read3 : DataStoreRead  Priority=1  DataStoreName=TqInpDetnStg2CenFilSt1
      settings: AttributesFormatString=priority: %<Priority>
  Data Store Read4 : DataStoreRead  Priority=1  DataStoreName=TqInpDetnStg2CenFilSt2
  Data Store Read5 : DataStoreRead  Priority=2  DataStoreName=TqInpDetnStg2CenFilSt1
      settings: AttributesFormatString=priority: %<Priority>
  Data Store Read6 : DataStoreRead  Priority=1  DataStoreName=TqInpDetnStg2UpFilSt1
      settings: AttributesFormatString=priority: %<Priority>
  Data Store Read7 : DataStoreRead  Priority=1  DataStoreName=TqInpDetnStg2UpFilSt2
  Data Store Read8 : DataStoreRead  Priority=2  DataStoreName=TqInpDetnStg2UpFilSt1
      settings: AttributesFormatString=priority: %<Priority>
  Data Store Write : DataStoreWrite  Priority=3  DataStoreName=TqInpDetnStg2DwnFilSt1
      settings: AttributesFormatString=priority: %<Priority>
  Data Store Write1 : DataStoreWrite  Priority=2  DataStoreName=TqInpDetnStg2DwnFilSt2
      settings: AttributesFormatString=priority: %<Priority>
  Data Store Write2 : DataStoreWrite  Priority=3  DataStoreName=TqInpDetnStg2CenFilSt1
      settings: AttributesFormatString=priority: %<Priority>
  Data Store Write3 : DataStoreWrite  Priority=2  DataStoreName=TqInpDetnStg2CenFilSt2
      settings: AttributesFormatString=priority: %<Priority>
  Data Store Write4 : DataStoreWrite  Priority=3  DataStoreName=TqInpDetnStg2UpFilSt1
      settings: AttributesFormatString=priority: %<Priority>
  Data Store Write5 : DataStoreWrite  Priority=2  DataStoreName=TqInpDetnStg2UpFilSt2
      settings: AttributesFormatString=priority: %<Priority>
  Goertzel_Part1_1 : Subsystem  TreatAsAtomicUnit=on
      settings: RTWSystemCode=Inline
  Goertzel_Part1_2 : Subsystem  TreatAsAtomicUnit=on
      settings: RTWSystemCode=Inline
  Goertzel_Part1_3 : Subsystem  TreatAsAtomicUnit=on
      settings: RTWSystemCode=Inline
  Subsystem5 : Subsystem  Description=|  mask(Copyright Information){none=on}
      | Copyright info block.                                               
      |                                                                     
      | Place copyright information at the top of every subsystem in design.
      mask prompts: none "No parameters"
      mask help: Place copyright information at the top of every subsystem in design.
      mask Display:
      | NxtrConf = 'Nexteer Confidential';
      | 
      | sys = bdroot; %handle for the current model ("system")
      | first = get_param(sys,'Created');
      | first = first(end-3:end);  %year is last four digits
      | 
      | last = get_param(sys,'LastModifiedDate');
      | if isempty(last)
      |     last = datestr(now,'yyyy');
      | else
      |     last = last(end-3:end);
      | end
      | 
      | if strcmp(first,last)
      |     fprintf('%s -- Copyright %s Nexteer',NxtrConf,first)
      | else
      |     fprintf('%s -- %s%s- %s Nexteer',NxtrConf,char(169),first,last)
      | end
  FrqDwnS0 : Outport
  FrqDwnS1 : Outport  Port=2
  FrqCenS0 : Outport  Port=3
  FrqCenS1 : Outport  Port=4
  FrqUpS0 : Outport  Port=5
  FrqUpS1 : Outport  Port=6
  wires:
  Stg1Outp/1 -> Goertzel_Part1_3/1(X0), Goertzel_Part1_2/1(X0), Goertzel_Part1_1/1(X0)
  Goertzel_Part1_1/1(S0) -> FrqDwnS0/1, Data Store Write/1  "FrqDwnFilSt0"
  Data Store Read1/1 -> Goertzel_Part1_1/3(S2)
  Constant2/1 -> Goertzel_Part1_1/2(FilGain)
  Data Store Read2/1 -> Data Store Write1/1
  Data Store Read/1 -> FrqDwnS1/1, Goertzel_Part1_1/4(S1)  "FrqDwnFiltSt1"
  Goertzel_Part1_2/1(S0) -> FrqCenS0/1, Data Store Write2/1  "FrqCenFilSt0"
  Data Store Read4/1 -> Goertzel_Part1_2/3(S2)
  Constant3/1 -> Goertzel_Part1_2/2(FilGain)
  Data Store Read5/1 -> Data Store Write3/1
  Data Store Read3/1 -> FrqCenS1/1, Goertzel_Part1_2/4(S1)  "FrqCenFilSt1"
  Goertzel_Part1_3/1(S0) -> FrqUpS0/1, Data Store Write4/1  "FrqUpFilSt0"
  Data Store Read7/1 -> Goertzel_Part1_3/3(S2)
  Constant4/1 -> Goertzel_Part1_3/2(FilGain)
  Data Store Read8/1 -> Data Store Write5/1
  Data Store Read6/1 -> FrqUpS1/1, Goertzel_Part1_3/4(S1)  "FrqUpFilSt1"

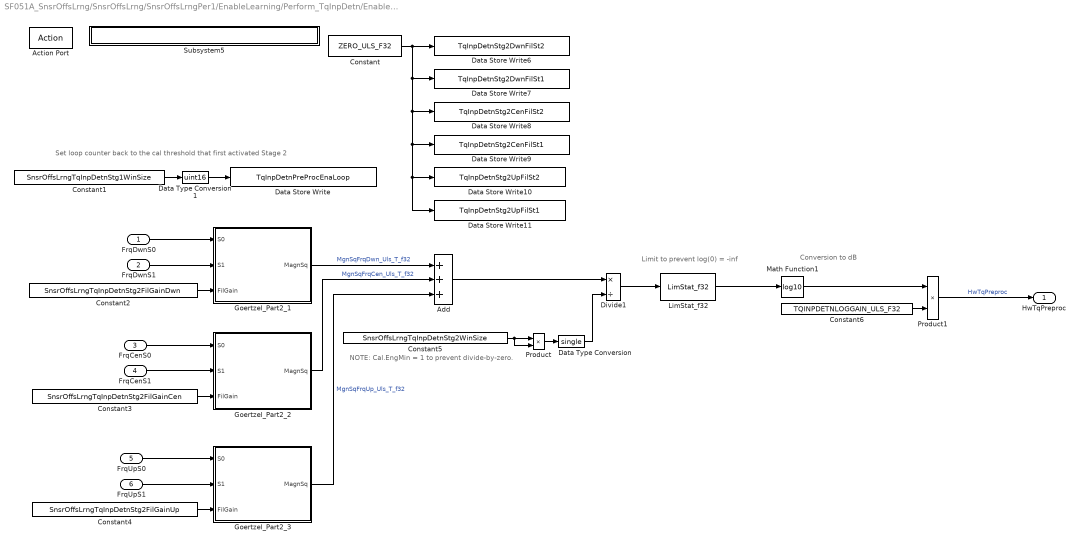
== system SF051A_SnsrOffsLrng/SnsrOffsLrng/SnsrOffsLrngPer1/EnableLearning/Perform_TqInpDetn/Enable_PreProcessing/Preprocessing/NewOut_ResetCntr ==
  note: NOTE: Cal.EngMin = 1 to prevent divide-by-zero.
  note: Set loop counter back to the cal threshold that first activated Stage 2
  note: Conversion to dB
  note: Limit to prevent log(0) = -inf
  FrqDwnS0 : Inport
  FrqDwnS1 : Inport  Port=2
  FrqCenS0 : Inport  Port=3
  FrqCenS1 : Inport  Port=4
  FrqUpS0 : Inport  Port=5
  FrqUpS1 : Inport  Port=6
  Action Port : ActionPort  ActionType=else
  Add : Sum  Inputs=+++
  Constant : Constant  Value=ZERO_ULS_F32  OutDataTypeStr=single
      settings: AttributesFormatString=%<OutDataTypeStr>
  Constant1 : Constant  Value=SnsrOffsLrngTqInpDetnStg1WinSize
  Constant2 : Constant  Value=SnsrOffsLrngTqInpDetnStg2FilGainDwn
  Constant3 : Constant  Value=SnsrOffsLrngTqInpDetnStg2FilGainCen
  Constant4 : Constant  Value=SnsrOffsLrngTqInpDetnStg2FilGainUp
  Constant5 : Constant  Value=SnsrOffsLrngTqInpDetnStg2WinSize
  Constant6 : Constant  Value=TQINPDETNLOGGAIN_ULS_F32
  Data Store Write : DataStoreWrite  DataStoreName=TqInpDetnPreProcEnaLoop
  Data Store Write10 : DataStoreWrite  DataStoreName=TqInpDetnStg2UpFilSt2
  Data Store Write11 : DataStoreWrite  DataStoreName=TqInpDetnStg2UpFilSt1
  Data Store Write6 : DataStoreWrite  DataStoreName=TqInpDetnStg2DwnFilSt2
  Data Store Write7 : DataStoreWrite  DataStoreName=TqInpDetnStg2DwnFilSt1
  Data Store Write8 : DataStoreWrite  DataStoreName=TqInpDetnStg2CenFilSt2
  Data Store Write9 : DataStoreWrite  DataStoreName=TqInpDetnStg2CenFilSt1
  Data Type Conversion : DataTypeConversion  OutDataTypeStr=single
  Data Type Conversion1 : DataTypeConversion  OutDataTypeStr=uint16
  Divide1 : Product  Inputs=*/
  Goertzel_Part2_1 : Subsystem  TreatAsAtomicUnit=on
      settings: RTWSystemCode=Inline
  Goertzel_Part2_2 : Subsystem  TreatAsAtomicUnit=on
      settings: RTWSystemCode=Inline
  Goertzel_Part2_3 : Subsystem  TreatAsAtomicUnit=on
      settings: RTWSystemCode=Inline
  LimStat_f32 : NxtrLim/LimStat_f32  LoLim=TQINPDETNLOGINPLOLIM_ULS_F32  HiLim=TQINPDETNLOGINPHILIM_ULS_F32
      settings: AttributesFormatString=|
      | Low Limit: %<LoLim>
      | High Limit:%<HiLim>
  Math Function1 : Math  Operator=log10  OutputSignalType=real  SaturateOnIntegerOverflow=on
  Product : Product
  Product1 : Product
  Subsystem5 : Subsystem  Description=|  mask(Copyright Information){none=on}
      | Copyright info block.                                               
      |                                                                     
      | Place copyright information at the top of every subsystem in design.
      mask prompts: none "No parameters"
      mask help: Place copyright information at the top of every subsystem in design.
      mask Display:
      | NxtrConf = 'Nexteer Confidential';
      | 
      | sys = bdroot; %handle for the current model ("system")
      | first = get_param(sys,'Created');
      | first = first(end-3:end);  %year is last four digits
      | 
      | last = get_param(sys,'LastModifiedDate');
      | if isempty(last)
      |     last = datestr(now,'yyyy');
      | else
      |     last = last(end-3:end);
      | end
      | 
      | if strcmp(first,last)
      |     fprintf('%s -- Copyright %s Nexteer',NxtrConf,first)
      | else
      |     fprintf('%s -- %s%s- %s Nexteer',NxtrConf,char(169),first,last)
      | end
  HwTqPreproc : Outport
  wires:
  Constant1/1 -> Data Type Conversion1/1
  Goertzel_Part2_2/1(MagnSq) -> Add/2  "MgnSqFrqCen_Uls_T_f32"
  Goertzel_Part2_3/1(MagnSq) -> Add/3  "MgnSqFrqUp_Uls_T_f32"
  Goertzel_Part2_1/1(MagnSq) -> Add/1  "MgnSqFrqDwn_Uls_T_f32"
  Product1/1 -> HwTqPreproc/1  "HwTqPreproc"
  FrqDwnS1/1 -> Goertzel_Part2_1/2(S1)
  FrqDwnS0/1 -> Goertzel_Part2_1/1(S0)
  FrqCenS1/1 -> Goertzel_Part2_2/2(S1)
  FrqCenS0/1 -> Goertzel_Part2_2/1(S0)
  FrqUpS1/1 -> Goertzel_Part2_3/2(S1)
  FrqUpS0/1 -> Goertzel_Part2_3/1(S0)
  Constant2/1 -> Goertzel_Part2_1/3(FilGain)
  Constant3/1 -> Goertzel_Part2_2/3(FilGain)
  Constant4/1 -> Goertzel_Part2_3/3(FilGain)
  Math Function1/1 -> Product1/1
  Add/1 -> Divide1/1
  Product/1 -> Data Type Conversion/1
  Divide1/1 -> LimStat_f32/1
  Constant5/1 -> Product/2, Product/1
  Data Type Conversion/1 -> Divide1/2
  Constant6/1 -> Product1/2
  Constant/1 -> Data Store Write11/1, Data Store Write10/1, Data Store Write9/1, Data Store Write8/1, Data Store Write7/1, Data Store Write6/1
  LimStat_f32/1 -> Math Function1/1
  Data Type Conversion1/1 -> Data Store Write/1
